simulink model "validateUSV"  (R2021a)
settings: Solver=FixedStepAuto  StartTime=0.0  StopTime=inf  FixedStep=SampleTime  RelTol=1e-3
values from neighbouring files (symbols this model uses):
  desideredSpeeds = 0:speedStep:maxSpeed    [identificateUSV.m]
  desideredYawRates = minYawRate:yawRateStep:maxYawRate    [identificateUSV.m]
  FFspeedCommands = interp1([0 speedMeanLevelSteps maxSpeed],                           [0 speedCommandLevelSteps 100],                            desideredSpeeds, 'pchip')    [identificateUSV.m]
  FFyawRateCommands = interp1([0 yawRateMeanLevelStepsFixed minYawRate maxYawRate],                            [0 yawRateCommandLevelStepsFixed -100 100],                            desideredYawRates, 'pchip')    [identificateUSV.m]
  lateralP1D = procest(idData,'P1D')    [identificateUSV.m]
  longitudinalP1D = procest(idData,'P1D')    [identificateUSV.m]
undefined symbols (not defined in the file or in its folder): USV
libraries: simulink x2
settings Model: EnablePacing=on  PacingRate=10  Creator=frank  LastModifiedBy=frank

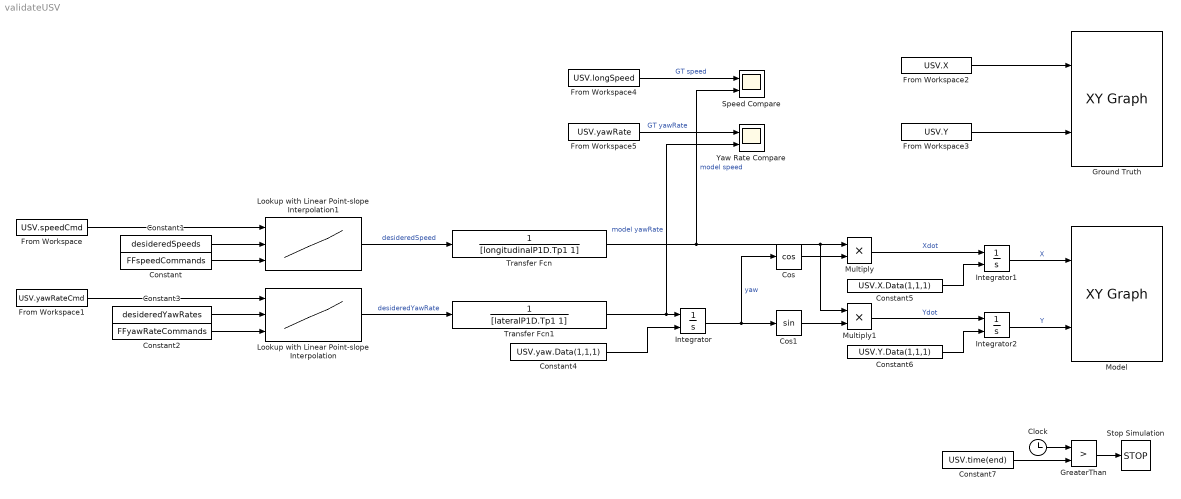
== system validateUSV ==
  Clock : Clock
  Constant : Constant  Value=FFspeedCommands
  Constant1 : Constant  Value=desideredSpeeds
  Constant2 : Constant  Value=FFyawRateCommands
  Constant3 : Constant  Value=desideredYawRates
  Constant4 : Constant  Value=USV.yaw.Data(1,1,1)
  Constant5 : Constant  Value=USV.X.Data(1,1,1)
  Constant6 : Constant  Value=USV.Y.Data(1,1,1)
  Constant7 : Constant  Value=USV.time(end)
  Cos : Trigonometry  Operator=cos
  Cos1 : Trigonometry
  From Workspace : FromWorkspace  VariableName=USV.speedCmd  OutputAfterFinalValue=Setting to zero
  From Workspace1 : FromWorkspace  VariableName=USV.yawRateCmd  OutputAfterFinalValue=Setting to zero
  From Workspace2 : FromWorkspace  VariableName=USV.X  OutputAfterFinalValue=Setting to zero
  From Workspace3 : FromWorkspace  VariableName=USV.Y  OutputAfterFinalValue=Setting to zero
  From Workspace4 : FromWorkspace  VariableName=USV.longSpeed  OutputAfterFinalValue=Setting to zero
  From Workspace5 : FromWorkspace  VariableName=USV.yawRate  OutputAfterFinalValue=Setting to zero
  GreaterThan : RelationalOperator  Operator=>  OutDataTypeStr=boolean  RndMeth=Simplest
  Ground Truth : simulink/Sinks/XY Graph  xmin=-340  xmax=-40  ymin=340  ymax=580  st=0.2
  Integrator : Integrator  InitialConditionSource=external
  Integrator1 : Integrator  InitialConditionSource=external
  Integrator2 : Integrator  InitialConditionSource=external
  Lookup with Linear Point-slope Interpolation : Lookup_n-D  NumberOfTableDimensions=1  BreakpointsForDimension1Source=Input port  BreakpointsForDimension1=[-5:5]  TableSource=Input port  Table=tanh([-5:5])  InternalRulePriority=Speed  RndMeth=Simplest  InputSameDT=on
      settings: InputPortMap=u0,p221,p5
  Lookup with Linear Point-slope Interpolation1 : Lookup_n-D  NumberOfTableDimensions=1  BreakpointsForDimension1Source=Input port  BreakpointsForDimension1=[-5:5]  TableSource=Input port  Table=tanh([-5:5])  InternalRulePriority=Speed  RndMeth=Simplest  InputSameDT=on
      settings: InputPortMap=u0,p221,p5
  Model : simulink/Sinks/XY Graph  xmin=-340  xmax=-40  ymin=340  ymax=580  st=0.2
  Multiply : Product  Inputs=**
  Multiply1 : Product  Inputs=**
  Speed Compare : Scope  NumInputPorts=2
  Stop Simulation : Stop
  Transfer Fcn : TransferFcn  Denominator=[longitudinalP1D.Tp1 1]
  Transfer Fcn1 : TransferFcn  Denominator=[lateralP1D.Tp1 1]
  Yaw Rate Compare : Scope  NumInputPorts=2
  wires:
  From Workspace/1 -> Lookup with Linear Point-slope Interpolation1/1
  Constant/1 -> Lookup with Linear Point-slope Interpolation1/3
  Constant1/1 -> Lookup with Linear Point-slope Interpolation1/2
  Lookup with Linear Point-slope Interpolation1/1 -> Transfer Fcn/1  "desideredSpeed"
  From Workspace1/1 -> Lookup with Linear Point-slope Interpolation/1
  Constant3/1 -> Lookup with Linear Point-slope Interpolation/2
  Constant2/1 -> Lookup with Linear Point-slope Interpolation/3
  Lookup with Linear Point-slope Interpolation/1 -> Transfer Fcn1/1  "desideredYawRate"
  Transfer Fcn1/1 -> Yaw Rate Compare/2, Integrator/1  "model yawRate"
  Integrator/1 -> Cos1/1, Cos/1  "yaw"
  Constant4/1 -> Integrator/2
  Transfer Fcn/1 -> Speed Compare/2, Multiply1/1, Multiply/1  "model speed"
  Cos/1 -> Multiply/2
  Cos1/1 -> Multiply1/2
  Multiply/1 -> Integrator1/1  "Xdot"
  Multiply1/1 -> Integrator2/1  "Ydot"
  Constant5/1 -> Integrator1/2
  Constant6/1 -> Integrator2/2
  Integrator1/1 -> Model/1  "X"
  Integrator2/1 -> Model/2  "Y"
  Clock/1 -> GreaterThan/1
  Constant7/1 -> GreaterThan/2
  GreaterThan/1 -> Stop Simulation/1
  From Workspace2/1 -> Ground Truth/1
  From Workspace3/1 -> Ground Truth/2
  From Workspace4/1 -> Speed Compare/1  "GT speed"
  From Workspace5/1 -> Yaw Rate Compare/1  "GT yawRate"
